simulink model "Roll_Diff_SS_D_1"  (R2013a)
settings: Solver=ode45  StartTime=0.0  StopTime=sim_length  RelTol=1e-3
values from neighbouring files (symbols this model uses):
  A_Roll_d = [1  0.02  0.00957373027909; 0  1  0.913912481482; 0  0  0.751477293075]    [Roll_Controller_SS_D_Data.mat]    (also in Roll_Controller_Sample_Time.m = A_d)
  B_Roll_d = [0.000933070289885 0.136767575416 0.248522706925]    [Roll_Controller_SS_D_Data.mat]    (also in Roll_Controller_Sample_Time.m = B_d)
  C_Roll_d = [1  0  0; 0  1  0]    [Roll_Controller_SS_D_Data.mat]    (also in Roll_Controller_Sample_Time.m = C_d)
  Feed_Forward_Roll_d = 0.125    [Roll_Controller_SS_D_Data.mat]    (also in Roll_Controller_Sample_Time.m)
  G_Roll_d = [0.251889913145  0.0200094814614; 0.229685260441  0.24715204306; -0.000711541775691  -9.30790483026e-05]    [Roll_Controller_SS_D_Data.mat]    (also in Roll_Controller_Sample_Time.m = place(A_d',C_d',P)')
  I_Theta = 0.122104044652    [Model_Parameters.mat]
  K_Roll_d = [2.67637429311 0.450684169535 1.07098831744]    [Roll_Controller_SS_D_Data.mat]    (also in Roll_Controller_Sample_Time.m = K_Roll_Reg(1:end-1))
  K_Roll_i = -2.24117965782    [Roll_Controller_SS_D_Data.mat]    (also in Roll_Controller_Sample_Time.m = K_Roll_Reg(end))
  Kf = 9.48907430341    [Model_Parameters.mat]
  L = 0.338    [Model_Parameters.mat]
  Motor_TimeConstant = 0.07    [Model_Parameters.mat]
  Ts = 20e-3    (= 0.02)    [All_Controller_Sample_Time.m]
undefined symbols (not defined in the file or in its folder): DiscIntNeverNeededParam
settings Model: Creator=Ross  LastModifiedBy=Ross

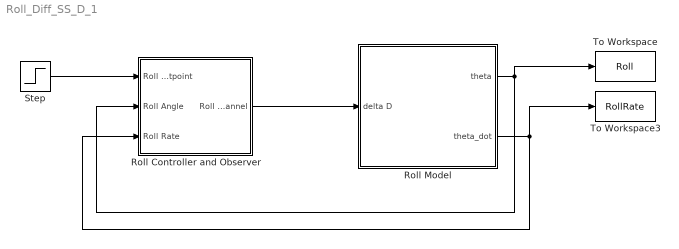
== system Roll_Diff_SS_D_1 ==
  Roll Controller and Observer : Subsystem
  Roll Model : Subsystem
  Step : Step  SampleTime=0
  To Workspace : ToWorkspace  VariableName=Roll  SampleTime=-1  SaveFormat=Timeseries
  To Workspace3 : ToWorkspace  VariableName=RollRate  SampleTime=-1  SaveFormat=Timeseries
  wires:
  Roll Model/1(theta) -> To Workspace/1, Roll Controller and Observer/2(Roll Angle)
  Roll Model/2(theta_dot) -> To Workspace3/1, Roll Controller and Observer/3(Roll Rate)
  Step/1 -> Roll Controller and Observer/1(Roll Setpoint)
  Roll Controller and Observer/1(Roll Channel) -> Roll Model/1(delta D)

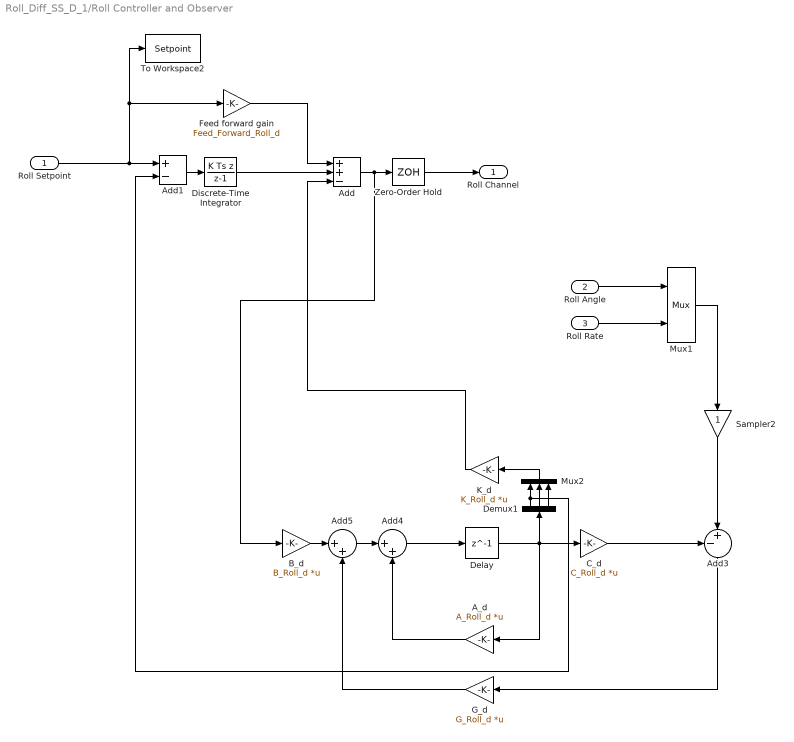
== system Roll_Diff_SS_D_1/Roll Controller and Observer ==
  Roll Setpoint : Inport
  Roll Angle : Inport  Port=2
  Roll Rate : Inport  Port=3
  A_d : Gain  Gain=A_Roll_d  Multiplication=Matrix(K*u)  SampleTime=Ts
  Add : Sum  Inputs=++-
  Add1 : Sum  Inputs=+-
  Add3 : Sum  Inputs=-+|
  Add4 : Sum  Inputs=|++
  Add5 : Sum  Inputs=|++
  "B_d " : Gain  Gain=B_Roll_d  Multiplication=Matrix(K*u)  SampleTime=Ts
  "C_d " : Gain  Gain=C_Roll_d  Multiplication=Matrix(K*u)  SampleTime=Ts
  Delay : Delay  DelayLength=1  InitialCondition=0  SampleTime=Ts
  Demux1 : Demux  Outputs=3
  Discrete-Time Integrator : DiscreteIntegrator  IntegratorMethod=Integration: Backward Euler  gainval=-K_Roll_i  SampleTime=Ts  ICPrevOutput=DiscIntNeverNeededParam  ICPrevScaledInput=DiscIntNeverNeededParam
  Feed forward gain : Gain  Gain=Feed_Forward_Roll_d  SampleTime=Ts
  G_d : Gain  Gain=G_Roll_d  Multiplication=Matrix(K*u)  SampleTime=Ts
  K_d : Gain  Gain=K_Roll_d  Multiplication=Matrix(K*u)  SampleTime=Ts
  Mux1 : Mux  Inputs=2
      settings: DisplayOption=signals
  Mux2 : Mux  Inputs=3
  Sampler2 : Gain  SampleTime=Ts
  To Workspace2 : ToWorkspace  VariableName=Setpoint  SampleTime=-1  SaveFormat=Timeseries
  Zero-Order Hold : ZeroOrderHold  SampleTime=Ts
  Roll Channel : Outport
  wires:
  Roll Rate/1 -> Mux1/2
  Roll Angle/1 -> Mux1/1
  Add5/1 -> Add4/1
  Demux1/3 -> Mux2/3
  Mux1/1 -> Sampler2/1
  G_d/1 -> Add5/2
  Demux1/2 -> Mux2/2
  A_d/1 -> Add4/2
  Add4/1 -> Delay/1
  "C_d "/1 -> Add3/1
  K_d/1 -> Add/3
  Sampler2/1 -> Add3/2
  Add/1 -> "B_d "/1, Zero-Order Hold/1
  "B_d "/1 -> Add5/1
  Demux1/1 -> Add1/2, Mux2/1
  Mux2/1 -> K_d/1
  Add3/1 -> G_d/1
  Delay/1 -> "C_d "/1, Demux1/1, A_d/1
  Zero-Order Hold/1 -> Roll Channel/1
  Discrete-Time Integrator/1 -> Add/2
  Roll Setpoint/1 -> To Workspace2/1, Feed forward gain/1, Add1/1
  Add1/1 -> Discrete-Time Integrator/1
  Feed forward gain/1 -> Add/1

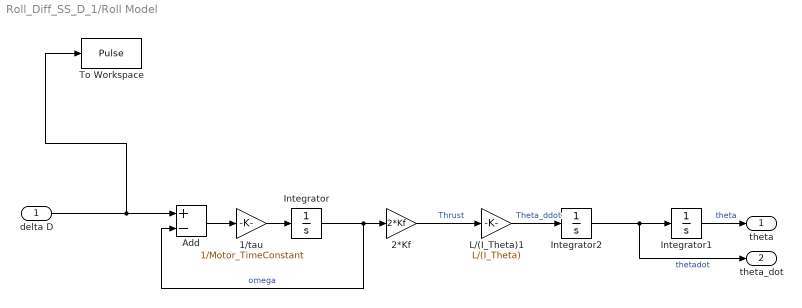
== system Roll_Diff_SS_D_1/Roll Model ==
  delta D : Inport
  1/tau : Gain  Gain=1/Motor_TimeConstant
  2*Kf : Gain  Gain=2*Kf
  Add : Sum  Inputs=+-
  Integrator : Integrator
  Integrator1 : Integrator
  Integrator2 : Integrator
  L/(I_Theta)1 : Gain  Gain=L/(I_Theta)
  To Workspace : ToWorkspace  VariableName=Pulse  SampleTime=-1  SaveFormat=Timeseries
  theta : Outport
  theta_dot : Outport  Port=2
  wires:
  2*Kf/1 -> L/(I_Theta)1/1  "Thrust"
  Integrator2/1 -> theta_dot/1, Integrator1/1  "thetadot"
  Add/1 -> 1/tau/1
  delta D/1 -> To Workspace/1, Add/1
  Integrator/1 -> 2*Kf/1, Add/2  "omega"
  1/tau/1 -> Integrator/1
  Integrator1/1 -> theta/1  "theta"
  L/(I_Theta)1/1 -> Integrator2/1  "Theta_ddot"
